simulink model "Mfunct1"  (R2020b)
settings: Solver=VariableStepAuto  StartTime=0.0  StopTime=30  RelTol=1e-3
libraries: simulink x1
settings Model: Creator=cesar  LastModifiedBy=cesar

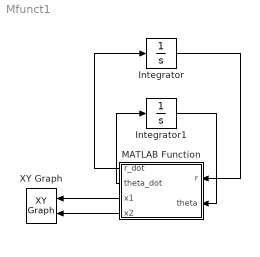
== system Mfunct1 ==
  Integrator : Integrator  InitialCondition=10
  Integrator1 : Integrator  InitialCondition=0.1
  MATLAB Function : MATLAB Function  TreatAsAtomicUnit=on
  XY Graph : simulink/Sinks/XY Graph  xmin=-3  xmax=15  ymin=-3  ymax=3  st=-1
  wires:
  Integrator/1 -> MATLAB Function/1(r)
  Integrator1/1 -> MATLAB Function/2(theta)
  MATLAB Function/1(r_dot) -> Integrator/1
  MATLAB Function/2(theta_dot) -> Integrator1/1
  MATLAB Function/3(x1) -> XY Graph/1
  MATLAB Function/4(x2) -> XY Graph/2

== matlab function Mfunct1/MATLAB Function ==
  data: r input; r_dot output; theta input; theta_dot output; x1 output; x2 output
function [r_dot, theta_dot, x1, x2] = fcn(r, theta)

r_dot = 0.05*r*(1-r);
theta_dot = (sin(theta/2))^2 ;

x1 = r*cos(theta);
x2 = r*sin(theta);
